simulink model "pr_wheel"  (R2024b)
settings: Solver=VariableStepAuto  StartTime=0.0  StopTime=20  RelTol=1e-3
values from neighbouring files (symbols this model uses):
  B_rw = [cos(alpha_rw), 0, -cos(alpha_rw), 0 ... (first row only)    [Parameter2.m]
  B_thr = [ 0,    0,    0,    0,   L_z, -L_z,  L_z, -L_z, -L_y,  L_y, -L_y,  L_y ... (first row only)    [Parameter2.m]
  D_thr = [ 1, 1,-1,-1,  0, 0, 0, 0,  0, 0, 0, 0 ... (first row only)    [Parameter2.m]
  sat_J = [0.288, 0, 0; 0, 0.45025, 0; 0, 0, 0.45025]    [Parameter2.m]
  sat_mass = 30    [Parameter2.m]
libraries: simulink x3
settings Model: Creator=10977  LastModifiedBy=10977

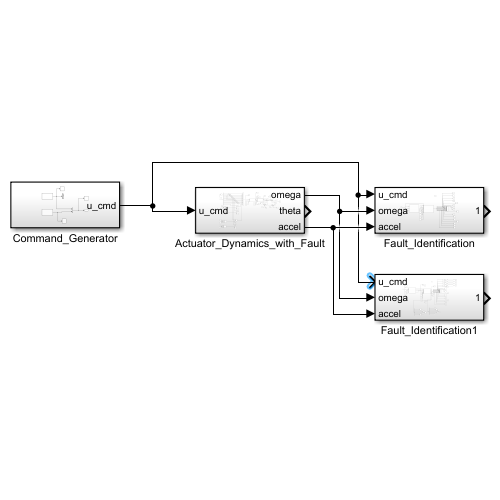
[thumbnail: Simulink's stored preview of the top-level diagram]
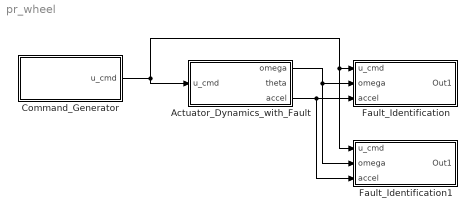
== system pr_wheel ==
  Actuator_Dynamics_with_Fault : Subsystem
  Command_Generator : Subsystem
  Fault_Identification : Subsystem
  Fault_Identification1 : Subsystem
  wires:
  Command_Generator/1(u_cmd) -> Fault_Identification1/1(u_cmd), Fault_Identification/1(u_cmd), Actuator_Dynamics_with_Fault/1(u_cmd)
  Actuator_Dynamics_with_Fault/1(omega) -> Fault_Identification1/2(omega), Fault_Identification/2(omega)
  Actuator_Dynamics_with_Fault/3(accel) -> Fault_Identification1/3(accel), Fault_Identification/3(accel)

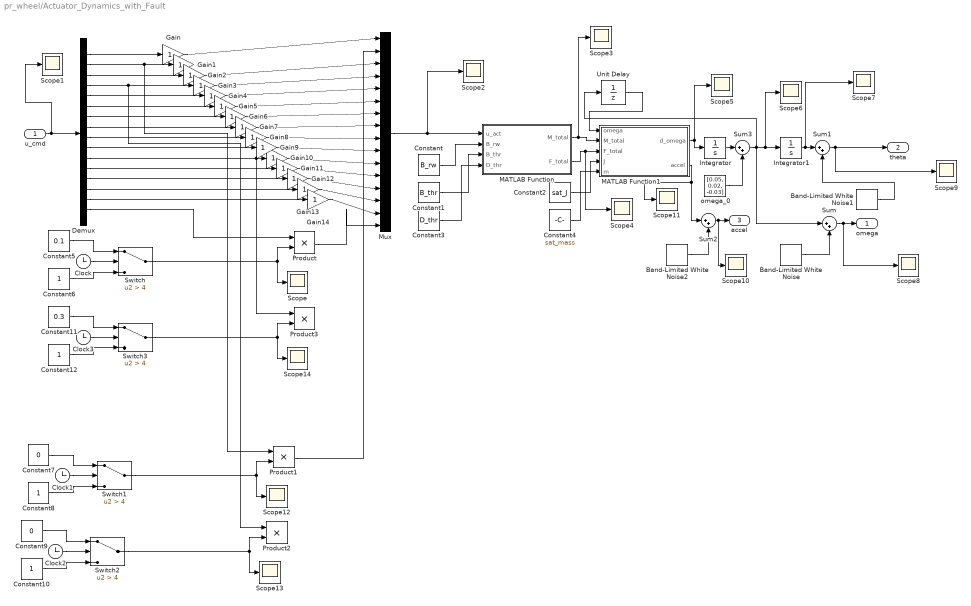
== system pr_wheel/Actuator_Dynamics_with_Fault ==
  u_cmd : Inport
  Band-Limited White Noise : simulink/Sources/Band-Limited White Noise  Cov=1e-10  Ts=0.01  seed=[23341]
  Band-Limited White Noise1 : simulink/Sources/Band-Limited White Noise  Cov=1e-8  Ts=0.01  seed=[23341]
  Band-Limited White Noise2 : simulink/Sources/Band-Limited White Noise  Cov=1e-10  Ts=0.01  seed=[26341]
  Clock{,1..3} (4 alike) : Clock
  Constant : Constant  Value=B_rw
  Constant1 : Constant  Value=B_thr
  Constant{6,8,10,12} (4 alike) : Constant
  Constant11 : Constant  Value=0.3
  Constant2 : Constant  Value=sat_J
  Constant3 : Constant  Value=D_thr
  Constant4 : Constant  Value=sat_mass
  Constant5 : Constant  Value=0.1
  Constant7 : Constant  Value=0
  Constant9 : Constant  Value=0
  Demux : Demux  Outputs=16
  Gain{,1..14} (15 alike) : Gain
  Integrator : Integrator
  Integrator1 : Integrator
  MATLAB Function : MATLAB Function  TreatAsAtomicUnit=on
  MATLAB Function1 : MATLAB Function  TreatAsAtomicUnit=on
  Mux : Mux  Inputs=16
  Product{,1..3} (4 alike) : Product
  Scope{,1..14} (15 alike) : Scope
  Sum{,1..3} (4 alike) : Sum  Inputs=|++
  Switch{,1..3} (4 alike) : Switch  Criteria=u2 > Threshold  Threshold=4  SaturateOnIntegerOverflow=off  InputSameDT=off
  Unit Delay : UnitDelay  InitialCondition=zeros(3,1)  SampleTime=0.01  HasFrameUpgradeWarning=on
  omega_0 : Constant  Value=[0.05, 0.02, -0.03]
  omega : Outport
  theta : Outport  Port=2
  accel : Outport  Port=3
  wires:
  u_cmd/1 -> Scope1/1, Demux/1
  Demux/2 -> Product1/1, Gain1/1
  Demux/3 -> Gain2/1
  Demux/4 -> Product2/1, Gain3/1
  Demux/5 -> Gain4/1
  Demux/6 -> Gain5/1
  Demux/7 -> Gain6/1
  Demux/8 -> Gain7/1
  Demux/9 -> Gain8/1
  Demux/10 -> Gain9/1
  Demux/11 -> Product3/1, Gain10/1
  Demux/12 -> Gain11/1
  Demux/13 -> Gain12/1
  Demux/14 -> Gain13/1
  Demux/15 -> Gain14/1
  Demux/16 -> Product/1
  Gain2/1 -> Mux/3
  Gain4/1 -> Mux/5
  Gain5/1 -> Mux/6
  Gain6/1 -> Mux/7
  Gain7/1 -> Mux/8
  Gain9/1 -> Mux/10
  Gain11/1 -> Mux/12
  Gain12/1 -> Mux/13
  Gain14/1 -> Mux/15
  Constant/1 -> MATLAB Function/2(B_rw)
  Constant1/1 -> MATLAB Function/3(B_thr)
  MATLAB Function/1(M_total) -> Scope3/1, MATLAB Function1/2(M_total)
  MATLAB Function1/1(d_omega) -> Scope5/1, Integrator/1
  Sum3/1 -> Sum/1, Unit Delay/1, Integrator1/1, Scope6/1
  Constant2/1 -> MATLAB Function1/4(J)
  Band-Limited White Noise/1 -> Sum/2
  Sum/1 -> Scope8/1, omega/1
  Integrator1/1 -> Scope7/1, Sum1/1
  Sum1/1 -> Scope9/1, theta/1
  Band-Limited White Noise1/1 -> Sum1/2
  Unit Delay/1 -> MATLAB Function1/1(omega)
  Constant3/1 -> MATLAB Function/4(D_thr)
  MATLAB Function/2(F_total) -> MATLAB Function1/3(F_total), Scope4/1
  Constant4/1 -> MATLAB Function1/5(m)
  Sum2/1 -> Scope10/1, accel/1
  MATLAB Function1/2(accel) -> Sum2/1, Scope11/1
  Band-Limited White Noise2/1 -> Sum2/2
  Clock/1 -> Switch/2
  Constant5/1 -> Switch/1
  Constant6/1 -> Switch/3
  Switch/1 -> Scope/1, Product/2
  Integrator/1 -> Sum3/1
  omega_0/1 -> Sum3/2
  Clock1/1 -> Switch1/2
  Constant7/1 -> Switch1/1
  Switch1/1 -> Scope12/1, Product1/2
  Constant8/1 -> Switch1/3
  Gain13/1 -> Mux/14
  Demux/1 -> Gain/1
  Gain8/1 -> Mux/9
  Gain/1 -> Mux/1
  Mux/1 -> MATLAB Function/1(u_act), Scope2/1
  Constant10/1 -> Switch2/3
  Constant9/1 -> Switch2/1
  Switch2/1 -> Scope13/1, Product2/2
  Clock2/1 -> Switch2/2
  Gain3/1 -> Mux/4
  Constant11/1 -> Switch3/1
  Clock3/1 -> Switch3/2
  Constant12/1 -> Switch3/3
  Switch3/1 -> Product3/2, Scope14/1
  Product/1 -> Mux/16
  Gain10/1 -> Mux/11
  Product1/1 -> Mux/2

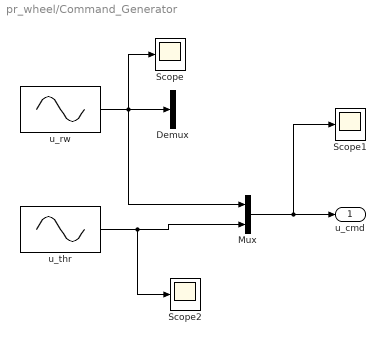
== system pr_wheel/Command_Generator ==
  Demux : Demux
  Mux : Mux  Inputs=2
  Scope : Scope
  Scope1 : Scope
  Scope2 : Scope
  u_rw : Sin  Amplitude=0.01  Frequency=2*pi*0.5  Phase=[0, pi/2, pi, 3*pi/2]  SampleTime=0.01
  u_thr : Sin  Amplitude=0.5  Frequency=2*pi*0.2  Phase=(0:11) * (2*pi/12)  SampleTime=0.01
  u_cmd : Outport
  wires:
  u_rw/1 -> Mux/1, Demux/1, Scope/1
  u_thr/1 -> Scope2/1, Mux/2
  Mux/1 -> u_cmd/1, Scope1/1

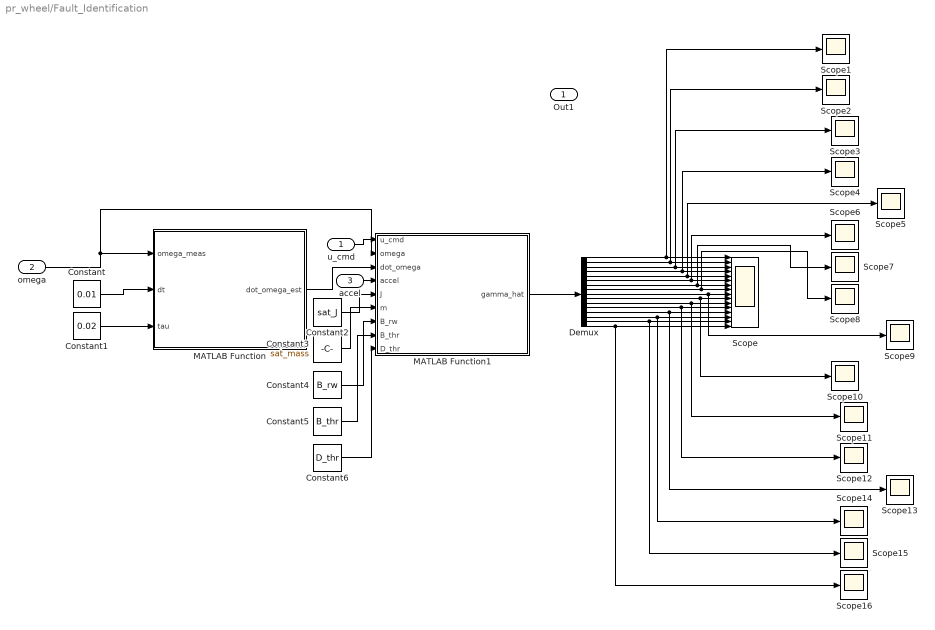
== system pr_wheel/Fault_Identification ==
  u_cmd : Inport
  omega : Inport  Port=2
  accel : Inport  Port=3
  Constant : Constant  Value=0.01
  Constant1 : Constant  Value=0.02
  Constant2 : Constant  Value=sat_J
  Constant3 : Constant  Value=sat_mass
  Constant4 : Constant  Value=B_rw
  Constant5 : Constant  Value=B_thr
  Constant6 : Constant  Value=D_thr
  Demux : Demux  Outputs=16
  MATLAB Function : MATLAB Function  TreatAsAtomicUnit=on  SystemSampleTime=0.01
  MATLAB Function1 : MATLAB Function  TreatAsAtomicUnit=on  SystemSampleTime=0.01
  Scope : Scope  NumInputPorts=16
  Scope{1..16} (16 alike) : Scope
  Out1 : Outport
  wires:
  omega/1 -> MATLAB Function1/2(omega), MATLAB Function/1(omega_meas)
  Constant/1 -> MATLAB Function/2(dt)
  Constant1/1 -> MATLAB Function/3(tau)
  u_cmd/1 -> MATLAB Function1/1(u_cmd)
  MATLAB Function/1(dot_omega_est) -> MATLAB Function1/3(dot_omega)
  Constant2/1 -> MATLAB Function1/5(J)
  MATLAB Function1/1(gamma_hat) -> Demux/1
  Demux/1 -> Scope1/1, Scope/1
  Demux/2 -> Scope2/1, Scope/2
  Demux/3 -> Scope3/1, Scope/3
  Demux/4 -> Scope4/1, Scope/4
  Demux/5 -> Scope5/1, Scope/5
  Demux/6 -> Scope6/1, Scope/6
  Demux/7 -> Scope7/1, Scope/7
  Demux/8 -> Scope8/1, Scope/8
  Demux/9 -> Scope9/1, Scope/9
  Demux/10 -> Scope10/1, Scope/10
  Demux/11 -> Scope11/1, Scope/11
  Demux/12 -> Scope12/1, Scope/12
  Demux/13 -> Scope13/1, Scope/13
  Demux/14 -> Scope14/1, Scope/14
  Demux/15 -> Scope15/1, Scope/15
  Demux/16 -> Scope16/1, Scope/16
  accel/1 -> MATLAB Function1/4(accel)
  Constant3/1 -> MATLAB Function1/6(m)
  Constant4/1 -> MATLAB Function1/7(B_rw)
  Constant5/1 -> MATLAB Function1/8(B_thr)
  Constant6/1 -> MATLAB Function1/9(D_thr)

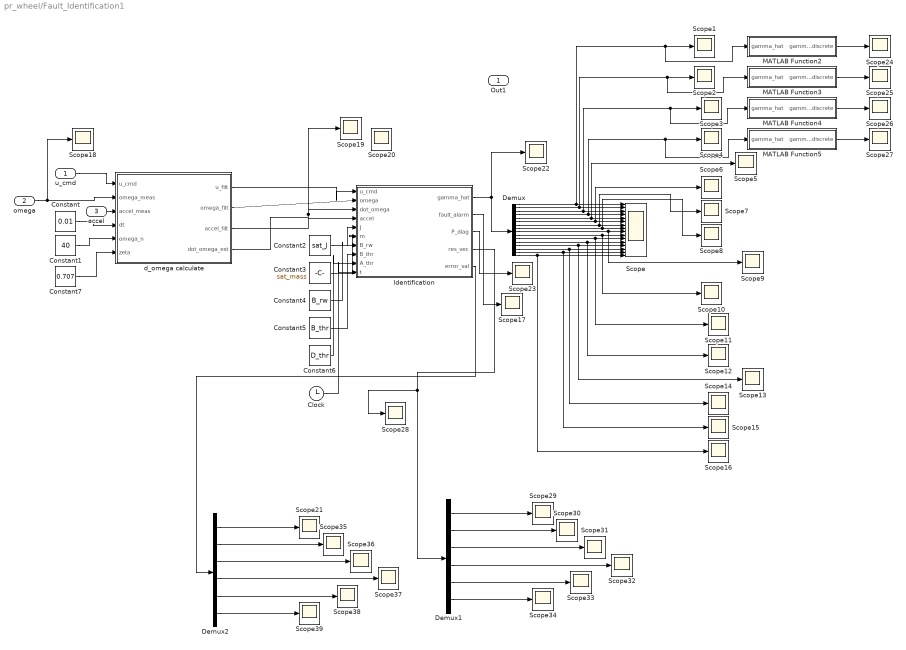
== system pr_wheel/Fault_Identification1 ==
  u_cmd : Inport
  omega : Inport  Port=2
  accel : Inport  Port=3
  Clock : Clock
  Constant : Constant  Value=0.01
  Constant1 : Constant  Value=40
  Constant2 : Constant  Value=sat_J
  Constant3 : Constant  Value=sat_mass
  Constant4 : Constant  Value=B_rw
  Constant5 : Constant  Value=B_thr
  Constant6 : Constant  Value=D_thr
  Constant7 : Constant  Value=0.707
  Demux : Demux  Outputs=16
  Demux1 : Demux  Outputs=6
  Demux2 : Demux  Outputs=6
  Identification : MATLAB Function  TreatAsAtomicUnit=on  SystemSampleTime=0.01
  MATLAB Function2 : MATLAB Function  TreatAsAtomicUnit=on  SystemSampleTime=0.01
  MATLAB Function3 : MATLAB Function  TreatAsAtomicUnit=on  SystemSampleTime=0.01
  MATLAB Function4 : MATLAB Function  TreatAsAtomicUnit=on  SystemSampleTime=0.01
  MATLAB Function5 : MATLAB Function  TreatAsAtomicUnit=on  SystemSampleTime=0.01
  Scope : Scope  NumInputPorts=16
  Scope{1..39} (39 alike) : Scope
  d_omega calculate : MATLAB Function  TreatAsAtomicUnit=on  SystemSampleTime=0.01
  Out1 : Outport
  wires:
  omega/1 -> Scope18/1, d_omega calculate/2(omega_meas)
  Constant/1 -> d_omega calculate/4(dt)
  Constant1/1 -> d_omega calculate/5(omega_n)
  d_omega calculate/4(dot_omega_est) -> Scope19/1, Identification/3(dot_omega)
  Constant2/1 -> Identification/5(J)
  Identification/1(gamma_hat) -> Demux/1, Scope22/1
  Demux/1 -> MATLAB Function2/1(gamma_hat), Scope1/1, Scope/1
  Demux/2 -> MATLAB Function3/1(gamma_hat), Scope2/1, Scope/2
  Demux/3 -> MATLAB Function4/1(gamma_hat), Scope3/1, Scope/3
  Demux/4 -> MATLAB Function5/1(gamma_hat), Scope4/1, Scope/4
  Demux/5 -> Scope5/1, Scope/5
  Demux/6 -> Scope6/1, Scope/6
  Demux/7 -> Scope7/1, Scope/7
  Demux/8 -> Scope8/1, Scope/8
  Demux/9 -> Scope9/1, Scope/9
  Demux/10 -> Scope10/1, Scope/10
  Demux/11 -> Scope11/1, Scope/11
  Demux/12 -> Scope12/1, Scope/12
  Demux/13 -> Scope13/1, Scope/13
  Demux/14 -> Scope14/1, Scope/14
  Demux/15 -> Scope15/1, Scope/15
  Demux/16 -> Scope16/1, Scope/16
  Constant3/1 -> Identification/6(m)
  Constant4/1 -> Identification/7(B_rw)
  Constant5/1 -> Identification/8(B_thr)
  Constant6/1 -> Identification/9(A_thr)
  Identification/2(fault_alarm) -> Scope17/1
  Clock/1 -> Identification/10(t)
  Identification/3(P_diag) -> Scope23/1
  Constant7/1 -> d_omega calculate/6(zeta)
  MATLAB Function2/1(gamma_discrete) -> Scope24/1
  MATLAB Function3/1(gamma_discrete) -> Scope25/1
  MATLAB Function4/1(gamma_discrete) -> Scope26/1
  MATLAB Function5/1(gamma_discrete) -> Scope27/1
  Identification/4(res_vec) -> Demux1/1, Scope28/1
  Demux1/1 -> Scope29/1
  Demux1/2 -> Scope30/1
  Demux1/3 -> Scope31/1
  Demux1/4 -> Scope32/1
  Demux1/5 -> Scope33/1
  Demux1/6 -> Scope34/1
  u_cmd/1 -> d_omega calculate/1(u_cmd)
  accel/1 -> d_omega calculate/3(accel_meas)
  d_omega calculate/1(u_filt) -> Identification/1(u_cmd)
  d_omega calculate/2(omega_filt) -> Identification/2(omega)
  d_omega calculate/3(accel_filt) -> Identification/4(accel)
  Demux2/2 -> Scope35/1
  Demux2/4 -> Scope37/1
  Demux2/3 -> Scope36/1
  Demux2/1 -> Scope21/1
  Identification/5(error_val) -> Demux2/1
  Demux2/5 -> Scope38/1
  Demux2/6 -> Scope39/1

== matlab function pr_wheel/Fault_Identification1/MATLAB Function2 ==
  data: gamma_hat input; gamma_discrete output
function gamma_discrete = fcn(gamma_hat)
    % gamma_hat: RLS辨识出的连续健康度 (16x1)
    % gamma_discrete: 输出的开关量 (16x1)
    
   
    
    % 对前4个飞轮执行硬化逻辑
    if gamma_hat >= 0.5
            gamma_discrete = 1.0;
        else
            gamma_discrete = 0.0;
    end
    
    
end

== matlab function pr_wheel/Fault_Identification1/MATLAB Function3 ==
  data: gamma_hat input; gamma_discrete output
function gamma_discrete = fcn(gamma_hat)
    % gamma_hat: RLS辨识出的连续健康度 (16x1)
    % gamma_discrete: 输出的开关量 (16x1)
    
   
    
    % 对前4个飞轮执行硬化逻辑
    if gamma_hat >= 0.5
            gamma_discrete = 1.0;
        else
            gamma_discrete = 0.0;
    end
    
    
end

== matlab function pr_wheel/Fault_Identification1/MATLAB Function4 ==
  data: gamma_hat input; gamma_discrete output
function gamma_discrete = fcn(gamma_hat)
    % gamma_hat: RLS辨识出的连续健康度 (16x1)
    % gamma_discrete: 输出的开关量 (16x1)
    
   
    
    % 对前4个飞轮执行硬化逻辑
    if gamma_hat >= 0.5
            gamma_discrete = 1.0;
        else
            gamma_discrete = 0.0;
    end
    
    
end

== matlab function pr_wheel/Fault_Identification1/MATLAB Function5 ==
  data: gamma_hat input; gamma_discrete output
function gamma_discrete = fcn(gamma_hat)
    % gamma_hat: RLS辨识出的连续健康度 (16x1)
    % gamma_discrete: 输出的开关量 (16x1)
    
   
    
    % 对前4个飞轮执行硬化逻辑
    if gamma_hat >= 0.5
            gamma_discrete = 1.0;
        else
            gamma_discrete = 0.0;
    end
    
    
end

== matlab function pr_wheel/Actuator_Dynamics_with_Fault/MATLAB Function1 ==
  data: omega input; M_total input; d_omega output; F_total input; J input; accel output; m input
function [d_omega, accel] = fcn(omega, M_total, F_total, J, m)
    % omega: 3x1 角速度
    % M_total: 3x1 合力矩
    % F_total: 3x1 合力 (新加)
    % J: 3x3 转动惯量
    % m: 卫星质量 (30kg)

    w = omega(:); 
    M = M_total(:);
    F = F_total(:);
    
    % 1. 姿态动力学 (计算角加速度)
    d_omega = J \ (M - cross(w, J * w));

    % 2. 轨道/平动动力学 (计算线加速度)
    % F = m * a  =>  a = F / m
    accel = F / m; 
end

== matlab function pr_wheel/Actuator_Dynamics_with_Fault/MATLAB Function ==
  data: u_act input; M_total output; B_rw input; B_thr input; D_thr input; F_total output
function [M_total, F_total] = fcn(u_act, B_rw, B_thr, D_thr)
    % u_act: 16维指令 (1-4飞轮, 5-16推进器)
    % B_rw: 3x4 飞轮力矩矩阵
    % B_thr: 3x12 推进器力矩矩阵
    % A_thr: 3x12 推进器推力矩阵 (新加)

    u_rw = u_act(1:4);
    u_thr = u_act(5:16);

    % 1. 合成三轴力矩 (飞轮 + 推进器)
    M_total = B_rw * u_rw + B_thr * u_thr;

    % 2. 合成三轴推力 (只有推进器产力)
    % 飞轮不产生任何平动推力，所以不参与计算
    F_total = D_thr * u_thr; 
end

== matlab function pr_wheel/Fault_Identification/MATLAB Function ==
  data: omega_meas input; dot_omega_est output; dt input; tau input
function dot_omega_est = fcn(omega_meas, dt, tau)
    % omega_meas: 带噪声的角速度观测值 (3x1)
    % dt: 仿真步长 (0.01s)
    % tau: 滤波时间常数 (建议设为 0.02 ~ 0.05)
    
    % 使用 persistent 变量存储上一时刻的状态实现离散化滤波
    persistent omega_prev dot_omega_prev
    
    if isempty(omega_prev)
        omega_prev = omega_meas;
        dot_omega_prev = [0; 0; 0];
    end
    
    % 离散化的一阶低通滤波微分公式 (基于后向差分)
    % 传递函数 G(s) = s / (tau*s + 1) 的离散化形式
    % alpha = tau / (tau + dt)
    alpha = tau / (tau + dt);
    
    % 计算当前时刻的角加速度估计值
    % 公式推导：y(k) = alpha * y(k-1) + (1 - alpha) * (u(k) - u(k-1)) / dt
    dot_omega_est = alpha * dot_omega_prev + (1 - alpha) * (omega_meas - omega_prev) / dt;
    
    % 更新状态供下一时刻使用
    omega_prev = omega_meas;
    dot_omega_prev = dot_omega_est;
end

== matlab function pr_wheel/Fault_Identification/MATLAB Function1 ==
  data: u_cmd input; gamma_hat output; omega input; dot_omega input; accel input; J input; m input; B_rw input; B_thr input; D_thr input
function gamma_hat = fcn(u_cmd, omega, dot_omega, accel, J, m, B_rw, B_thr, D_thr)
    % 输入新增：accel (3x1 线加速度), m (质量), A_thr (推力矩阵)
    
    persistent P theta_hat lambda
    num_act = 16;
    
    if isempty(P)
        P = eye(num_act) * 1e8; 
        theta_hat = ones(num_act, 1); 
        lambda = 0.985; 
    end

    %% 1. 构造 6 维观测向量 Y (3力矩 + 3力)
    % 姿态观测：M = J*dw + w x Jw
    M_meas = J * dot_omega + cross(omega, J * omega);
    % 平动观测：F = m * a
    F_meas = m * accel;
    
    % 合并成 6x1 观测向量
    Y = [M_meas; F_meas];

    %% 2. 构造 6x16 的增强回归矩阵 H
    % 上半部分 (1-3行)：力矩分配 [B_rw, B_thr]
    H_torque = [B_rw, B_thr];
    % 下半部分 (4-6行)：推力分配 [飞轮贡献为0, 推进器贡献为A_thr]
    H_force = [zeros(3,4), D_thr];
    
    % 最终回归矩阵 (考虑指令大小)
    H = [H_torque; H_force] * diag(u_cmd);

    %% 3. RLS 递推 (现在是在 6 维空间里找 16 个未知数)
    % K 现在是 16x6 的矩阵
    K = (P * H') / (lambda * eye(6) + H * P * H');
    
    error = Y - H * theta_hat;
    theta_hat = theta_hat + K * error;
    P = (P - K * H * P) / lambda;

    gamma_hat = theta_hat;
end

== matlab function pr_wheel/Fault_Identification1/d_omega calculate ==
  data: u_cmd input; u_filt output; omega_filt output; accel_filt output; omega_meas input; accel_meas input; dot_omega_est output; dt input; omega_n input; zeta input
function [u_filt, omega_filt, accel_filt, dot_omega_est] = fcn(u_cmd, omega_meas, accel_meas, dt, omega_n, zeta)
    % u_cmd: (16x1) 执行机构指令
    % omega_meas: (3x1) 角速度测量
    % accel_meas: (3x1) 加速度测量
    
    % 1. 为所有信号定义 persistent 状态 (x1为信号，x2为导数)
    persistent om_x1 om_x2 u_x1 u_x2 ac_x1 ac_x2
    
    % 2. 初始化 (首次运行时对齐初值，减少启动冲击)
    if isempty(om_x1)
        om_x1 = omega_meas;  om_x2 = zeros(3,1);
        u_x1  = u_cmd;       u_x2  = zeros(16,1);
        ac_x1 = accel_meas;  ac_x2 = zeros(3,1);
    end
    
    %% 核心算法：统一的二阶动力学滤波
    % 公式：ddy + 2*zeta*wn*dy + wn^2*y = wn^2*u
    % 这种写法的逻辑是：所有信号共享相同的 omega_n 和 zeta，保证相位滞后完全一致
    
    % --- 角速度与角加速度分支 ---
    err_om = om_x1 - omega_meas;
    dom_x1 = om_x2;
    dom_x2 = -omega_n^2 * err_om - 2*zeta*omega_n * om_x2;
    
    % --- 指令信号分支 (只取滤波值 x1) ---
    err_u = u_x1 - u_cmd;
    du_x1 = u_x2;
    du_x2 = -omega_n^2 * err_u - 2*zeta*omega_n * u_x2;
    
    % --- 加速度信号分支 (只取滤波值 x1) ---
    err_ac = ac_x1 - accel_meas;
    dac_x1 = ac_x2;
    dac_x2 = -omega_n^2 * err_ac - 2*zeta*omega_n * ac_x2;
    
    %% 3. 欧拉积分更新状态
    om_x1 = om_x1 + dom_x1 * dt;
    om_x2 = om_x2 + dom_x2 * dt;
    
    u_x1  = u_x1 + du_x1 * dt;
    u_x2  = u_x2 + du_x2 * dt;
    
    ac_x1 = ac_x1 + dac_x1 * dt;
    ac_x2 = ac_x2 + dac_x2 * dt;
    
    %% 4. 输出对齐后的信号
    % omega_filt 对应的是 om_x1，它的滞后量与 dot_omega_est (om_x2) 严格匹配
    omega_filt    = om_x1;
    dot_omega_est = om_x2;
    
    % u_filt 和 accel_filt 经历了同样的二阶低通过程
    u_filt     = u_x1;
    accel_filt = ac_x1;
end

== matlab function pr_wheel/Fault_Identification1/Identification ==
  data: u_cmd input; gamma_hat output; omega input; dot_omega input; accel input; J input; m input; B_rw input; B_thr input; A_thr input; fault_alarm output; t input; P_diag output; res_vec output; error_val output
function [gamma_hat, fault_alarm, P_diag, res_vec, error_val] = fcn(u_cmd, omega, dot_omega, accel, J, m, B_rw, B_thr, A_thr, t)
    % 显式声明外部函数，用于在 Simulink 仿真中打印调试信息
    coder.extrinsic('fprintf');
    
    % --- 变量说明 ---
    % 状态向量 theta_hat (16x1): 1-4位为飞轮健康度, 5-16位为推进器健康度 (1为正常, 0为完全失效)
    % P (16x16): 辨识协方差矩阵，代表对当前估计结果的“不确定性”
    % is_faulted: 故障标志位（一旦触发，锁定为1）
    % timer: 故障发生后的计时器（帧数），用于触发不同阶段的辨识策略
    % res_integral: 残差积分，用于消除辨识稳态误差
    persistent P theta_hat is_faulted timer res_integral
    
    %% 1. 初始化 (首次运行)
    if isempty(P)
        P = eye(16);
        P(1:4, 1:4) = eye(4) * 0.1;     % 初始状态下飞轮较为信任
        P(5:16, 5:16) = eye(12) * 0.01; % 初始状态下推进器较为信任
        theta_hat = ones(16, 1);        % 默认初始状态全健康
        is_faulted = 0;           
        timer = 0;   
        res_integral = zeros(6, 1);     % 初始积分项为0
    end

    %% 2. 观测模型构造 (物理模型映射)
    % 计算理论力矩 (Euler方程) 和 理论合外力
    M_meas = J * dot_omega + cross(omega, J * omega);
    F_meas = m * accel;
    Y = [M_meas; F_meas]; % 组合成 6x1 观测向量
    
    % 构造观测矩阵 H (将控制指令映射到力/力矩空间)
    % 前4列对应飞轮对力矩的影响, 后12列对应推进器对力/力矩的影响
    H_mat = [B_rw, B_thr; zeros(3,4), A_thr] * diag(u_cmd);
    
    % 默认辨识目标 Y_comp，初始化为原始观测
    Y_comp = Y; 
    
    % 计算“健康残差”：测量值与“假设全健康”模型之间的偏差
    res_for_alarm = Y - H_mat * ones(16,1); 
    res_vec = res_for_alarm; 
    
    % --- 故障检测逻辑 ---
    % t>0.5s 是为了避开启动冲击；若力矩或力残差超过阈值(0.01)，判定故障
    if t > 0.5 && is_faulted == 0
        if norm(res_for_alarm(1:3)) > 0.01 || norm(res_for_alarm(4:6)) > 0.01 
            is_faulted = 1;
        end
    end
    fault_alarm = is_faulted;

    %% 3. 唤醒层：突变响应与自适应学习率 (遗忘因子)
    lambda = 0.998; % 默认稳态遗忘因子，值越大系统越稳，值越小对新信息越敏感
    
    if is_faulted == 1
        if timer == 0
            % --- 故障爆发瞬间 (第0帧) ---
            % 使用伪逆进行“初值投影”，试图瞬间定位故障位置，跳过 RLS 漫长的爬升期
            delta_theta = pinv(H_mat) * res_for_alarm;
            theta_hat = ones(16, 1) + delta_theta;
            
            % 打印初值以便分析投影是否准确
            fprintf('\n--- [FDI Trigger] Initial Projection at %.3f s ---\n', t);
            for i = 1:16
                fprintf('Ch %d: %.3f | ', i, theta_hat(i));
                if mod(i,4)==0, fprintf('\n'); end
            end
            
            % 瞬间拉大协方差 P，表示此时对“全健康”假设彻底不信任，重启大规模搜索
            P = eye(16);
            P(1:4, 1:4) = eye(4) * 2000;    
            P(5:16, 5:16) = eye(12) * 1000; 
            lambda = 0.80; % 初始遗忘因子设小，允许参数剧烈跳变
            timer = 1; 
        else
            % --- 辨识过渡期 (持续运行) ---
            % 基于当前辨识残差计算 lambda
            res_est = Y - H_mat * theta_hat; 
            res_norm_est = norm(res_est);
            
            % 【关键逻辑：残差积分补偿】
            % 通过对残差积分并反馈到观测端，强行消除辨识过程中的静差，加速尾迹收敛
            Ki = 0.3; 
            res_integral = res_integral + res_est * 0.01; % dt = 0.01s
            Y_comp = Y + Ki * res_integral; 
            
            % 【关键逻辑：自适应 VFF 公式】
            % 当残差大时 lambda 自动变小（加速追赶）；残差小时 lambda 回升（锁定结果防止震荡）
            lambda = 0.82 + (0.999 - 0.82) * exp(-150 * res_norm_est^2);
            lambda = max(min(lambda, 0.999), 0.80);
            
            timer = timer + 1;
            fprintf('\nTime: %.3f, Lambda: %.4f \n', t, lambda);
        end
    end

    %% 4. 收敛层：硬化保护与加权递归最小二乘 (RLS)
    theta_internal = theta_hat;
    
    % --- 飞轮硬化逻辑 ---
    % 故障 0.25s 后，若飞轮健康度辨识值 > 0.5，强制判定为 1 (健康)
    % 理由：飞轮故障概率低且通常具有确定性，硬化可以防止飞轮与推进器之间产生参数耦合干扰
    if timer > 25
        for i = 1:4
            theta_internal(i) = (theta_hat(i) > 0.5); 
        end
    end

    % 计算辨识误差 (使用带积分补偿的 Y_comp)
    error_val = Y_comp - H_mat * theta_internal; 
    
    % --- 通道加权矩阵 W ---
    % w_accel 设置为 50，意味着“合外力/加速度”通道的误差权重要比“力矩”通道大 50 倍
    % 效果：强迫辨识器优先匹配推进器引起的长周期加速度偏差
    w_accel = 50; 
    W_vec = [1; 1; 1; w_accel; w_accel; w_accel];
    W_mat = diag(W_vec);
    
    % --- 标准 RLS 迭代更新 (带加权 W) ---
    PHt = P * H_mat';
    % 计算增益矩阵 K
    K = (PHt * W_mat) / (lambda * eye(6) + H_mat * PHt * W_mat);
    
    % 更新估计值 theta_hat
    theta_hat = theta_hat + K * error_val;
    % 更新协方差矩阵 P (Joseph 形式简化)
    P = (P - K * H_mat * P) / lambda;

    %% 5. 输出限制与映射
    % 限制 theta 在有效物理范围内 (0 到 1.2, 1.2 留出一点超调余量)
    gamma_hat = max(min(theta_hat, 1.2), 0);
    P_diag = diag(P); % 输出 P 阵对角线，用于监测算法收敛置信度
end
